simulink model "withshapingprgmdistsim"  (Simulink 6.3)
settings: Solver=ode45  StartTime=0.0  StopTime=60  RelTol=1e-3
values from neighbouring files (symbols this model uses):
  A = [  -0.1778         0         0         0         0   -9.7807   -9.7807 ... (first row only)    [shapingprgmdist.m]    (also in shapingprgmdist_withsigma.m)
  Aw = [-1/tauc 0; 0 -1/tauc]    [shapingprgmdist.m]    (also in shapingprgmdist_withsigma.m)
  B = [B1(:,1) B1(:,2) B1(:,4)]    [shapingprgmdist.m]    (also in shapingprgmdist_withsigma.m)
  Bw = .5*eye(2)    [shapingprgmdist.m]    (also in shapingprgmdist_withsigma.m)
  C = zeros(5,11)    [shapingprgmdist.m]    (also in shapingprgmdist_withsigma.m)
  D = [(W1G.a(:,1)) (W1G.a(:,2))]    [shapingprgmdist.m]    (also in shapingprgmdist_withsigma.m)
  den11 = [1 5 0]    [shapingprgmdist.m]    (also in shapingprgmdist_withsigma.m)
  den22 = den11    [shapingprgmdist.m]    (also in shapingprgmdist_withsigma.m)
  den33 = den11    [shapingprgmdist.m]    (also in shapingprgmdist_withsigma.m)
  K = inv(R)*(B'*P)*C'*inv(C*C')    [Hinfopfb.m]    (also in shapingprgmdist.m = Hinfopfb(W1G.a,W1G.b,W1G.c,D,gamma,Q,R); shapingprgmdist_withsigma.m = Hinfopfb(W1G.a,W1G.b,W1G.c,D,gamma,Q,R))
  num11 = 3*[1 0.5]    [shapingprgmdist.m]    (also in shapingprgmdist_withsigma.m)
  num22 = num11    [shapingprgmdist.m]    (also in shapingprgmdist_withsigma.m)
  num33 = num11    [shapingprgmdist.m]    (also in shapingprgmdist_withsigma.m)
  Phicorr = 1    [shapingprgmdist.m]    (also in shapingprgmdist_withsigma.m)
  qu = -20*0.3048    (= -6.096)    [shapingprgmdist.m]    (also in shapingprgmdist_withsigma.m)
  qv = -20*0.3048    (= -6.096)    [shapingprgmdist.m]    (also in shapingprgmdist_withsigma.m)
  Thetacorr = 1    [shapingprgmdist.m]    (also in shapingprgmdist_withsigma.m)
  W2 = diag([1 1 1 1 1])    [shapingprgmdist.m]    (also in shapingprgmdist_withsigma.m)
libraries: simulink x1
settings Model: LastModifiedBy=JG

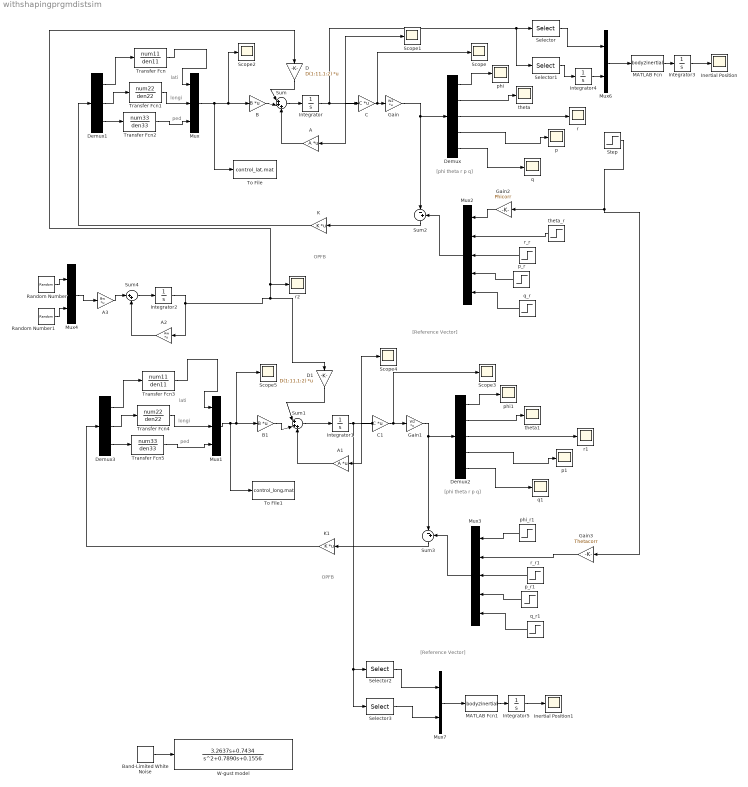
== system withshapingprgmdistsim ==
  note: OPFB
  note: [phi theta r p q]
  note: lati
  note: longi
  note: ped
  note: [Reference Vector]
  note: OPFB
  note: [phi theta r p q]
  note: [Reference Vector]
  note: lati
  note: longi
  note: ped
  A : Gain  Orientation=left  Gain=A  Multiplication=Matrix(K*u)
  A1 : Gain  Orientation=left  Gain=A  Multiplication=Matrix(K*u)
  A2 : Gain  Orientation=left  Gain=Aw  Multiplication=Matrix(K*u)
  A3 : Gain  Gain=Bw  Multiplication=Matrix(K*u)
  B : Gain  Gain=B  Multiplication=Matrix(K*u)
  B1 : Gain  Gain=B  Multiplication=Matrix(K*u)
  Band-Limited White Noise : simulink/Sources/Band-Limited White Noise  Cov=.1  Ts=0.1  seed=[23341]
  C : Gain  Gain=C  Multiplication=Matrix(K*u)
  C1 : Gain  Gain=C  Multiplication=Matrix(K*u)
  D : Gain  Orientation=down  Gain=D(1:11,1:2)  Multiplication=Matrix(K*u)
  D1 : Gain  Orientation=down  Gain=D(1:11,1:2)  Multiplication=Matrix(K*u)
  Demux : Demux  Outputs=5
  Demux1 : Demux  Outputs=3
  Demux2 : Demux  Outputs=5
  Demux3 : Demux  Outputs=3
  Gain : Gain  Gain=W2  Multiplication=Matrix(K*u)
  Gain1 : Gain  Gain=W2  Multiplication=Matrix(K*u)
  Gain2 : Gain  Orientation=left  Gain=Phicorr
  Gain3 : Gain  Orientation=left  Gain=Thetacorr
  Inertial Position : Scope
      settings: SaveName=InertialPos  DataFormat=Array
  Inertial Position1 : Scope
      settings: SaveName=InertialPos1  DataFormat=Array
  Integrator : Integrator  InitialCondition=rand((size(A,1)),1)*0.01
  Integrator1 : Integrator  InitialCondition=rand((size(A,1)),1)*0.01
  Integrator2 : Integrator
  Integrator3 : Integrator  InitialCondition=[0;0;-50]
  Integrator4 : Integrator
  Integrator5 : Integrator  InitialCondition=[0;0;-50]
  K : Gain  Orientation=left  Gain=K  Multiplication=Matrix(K*u)
  K1 : Gain  Orientation=left  Gain=K  Multiplication=Matrix(K*u)
  MATLAB Fcn : MATLABFcn  MATLABFcn=body2inertial
  MATLAB Fcn1 : MATLABFcn  MATLABFcn=body2inertial
  Mux : Mux  Inputs=3
  Mux1 : Mux  Inputs=3
  Mux2 : Mux  Orientation=left  Inputs=5
  Mux3 : Mux  Orientation=left  Inputs=5
  Mux4 : Mux  Inputs=2
  Mux6 : Mux  Inputs=2
  Mux7 : Mux  Inputs=2
  Random Number : RandomNumber  Variance=qu^2  SampleTime=0
  Random Number1 : RandomNumber  Variance=qv^2  Seed=5000  SampleTime=0
  Scope{,1..5} (6 alike) : Scope
      Scope settings: SaveName=y  DataFormat=Array
      Scope1 settings: SaveName=x1  DataFormat=Array
      Scope2 settings: SaveName=ScopeData8
      Scope3 settings: SaveName=y2  DataFormat=Array
      Scope4 settings: SaveName=x2  DataFormat=Array
  Selector : Selector  Elements=[1 2 9 5 6]  InputPortWidth=11
  Selector1 : Selector  Elements=[10]  InputPortWidth=11
  Selector2 : Selector  Elements=[1 2 9 5 6]  InputPortWidth=11
  Selector3 : Selector  Elements=10  InputPortWidth=11
  Step : Step  Time=0  SampleTime=0
  Sum : Sum  Inputs=|+++
  Sum1 : Sum  Inputs=|+++
  Sum2 : Sum  Orientation=down  Inputs=|-+
  Sum3 : Sum  Orientation=down  Inputs=|-+
  Sum4 : Sum  Inputs=|++
  To File : ToFile  Filename=control_lat.mat  MatrixName=ulat
  To File1 : ToFile  Filename=control_long.mat  MatrixName=ulong
  Transfer Fcn : TransferFcn  Numerator=num11  Denominator=den11
  Transfer Fcn1 : TransferFcn  Numerator=num22  Denominator=den22
  Transfer Fcn2 : TransferFcn  Numerator=num33  Denominator=den33
  Transfer Fcn3 : TransferFcn  Numerator=num11  Denominator=den11
  Transfer Fcn4 : TransferFcn  Numerator=num22  Denominator=den22
  Transfer Fcn5 : TransferFcn  Numerator=num33  Denominator=den33
  W-gust model : TransferFcn  Numerator="[3.2637    0.7434]"  Denominator="[1.0000    0.7890    0.1556]"
  p : Scope
      settings: SaveName=ScopeData4
  p1 : Scope
      settings: SaveName=ScopeData6
  p_r : Step  Orientation=left  Time=0  After=0  SampleTime=0
  p_r1 : Step  Orientation=left  Time=0  After=0  SampleTime=0
  phi : Scope
  phi1 : Scope
      settings: SaveName=ScopeData7
  phi_r1 : Step  Orientation=left  Time=0  After=0  SampleTime=0
  q : Scope
      settings: SaveName=ScopeData5
  q1 : Scope
      settings: SaveName=ScopeData9
  q_r : Step  Orientation=left  Time=0  After=0  SampleTime=0
  q_r1 : Step  Orientation=left  Time=0  After=0  SampleTime=0
  r : Scope
      settings: SaveName=ScopeData3
  r1 : Scope
      settings: SaveName=ScopeData10
  r2 : Scope
      settings: SaveName=d  DataFormat=Array
  r_r : Step  Orientation=left  Time=0  After=0  SampleTime=0
  r_r1 : Step  Orientation=left  Time=0  After=0  SampleTime=0
  theta : Scope
      settings: SaveName=ScopeData2
  theta1 : Scope
      settings: SaveName=ScopeData11
  theta_r : Step  Orientation=left  Time=0  After=0  SampleTime=0
  wires:
  Integrator/1 -> A/1, C/1, Scope1/1, Selector/1, Selector1/1
  Sum/1 -> Integrator/1
  C/1 -> Gain/1, Scope/1
  Mux/1 -> B/1, Scope2/1, To File/1
  Mux2/1 -> Sum2/2
  r_r/1 -> Mux2/3
  Sum2/1 -> K/1
  K/1 -> Demux1/1
  Demux/1 -> phi/1
  Demux/2 -> theta/1
  Demux/3 -> r/1
  Step/1 -> Gain2/1, Gain3/1
  theta_r/1 -> Mux2/2
  p_r/1 -> Mux2/4
  q_r/1 -> Mux2/5
  Demux/4 -> p/1
  Demux/5 -> q/1
  Integrator1/1 -> A1/1, C1/1, Scope4/1, Selector3/1, Selector2/1
  Sum1/1 -> Integrator1/1
  C1/1 -> Gain1/1, Scope3/1
  Mux1/1 -> B1/1, Scope5/1, To File1/1
  Mux3/1 -> Sum3/2
  r_r1/1 -> Mux3/3
  Sum3/1 -> K1/1
  K1/1 -> Demux3/1
  Demux2/1 -> phi1/1
  Demux2/2 -> theta1/1
  Demux2/3 -> r1/1
  phi_r1/1 -> Mux3/1
  p_r1/1 -> Mux3/4
  q_r1/1 -> Mux3/5
  Demux2/4 -> p1/1
  Demux2/5 -> q1/1
  Demux1/1 -> Transfer Fcn/1
  Demux1/3 -> Transfer Fcn2/1
  Demux1/2 -> Transfer Fcn1/1
  Transfer Fcn1/1 -> Mux/2
  Demux3/1 -> Transfer Fcn3/1
  Demux3/3 -> Transfer Fcn5/1
  Transfer Fcn5/1 -> Mux1/3
  Demux3/2 -> Transfer Fcn4/1
  Transfer Fcn4/1 -> Mux1/2
  Gain/1 -> Demux/1, Sum2/1
  Gain1/1 -> Demux2/1, Sum3/1
  Transfer Fcn2/1 -> Mux/3
  Gain2/1 -> Mux2/1
  Gain3/1 -> Mux3/2
  A/1 -> Sum/3
  B/1 -> Sum/2
  A1/1 -> Sum1/3
  B1/1 -> Sum1/2
  Transfer Fcn3/1 -> Mux1/1
  Transfer Fcn/1 -> Mux/1
  D/1 -> Sum/1
  D1/1 -> Sum1/1
  Band-Limited White Noise/1 -> W-gust model/1
  Integrator2/1 -> A2/1, D1/1, D/1, r2/1
  Random Number/1 -> Mux4/1
  Random Number1/1 -> Mux4/2
  A2/1 -> Sum4/2
  Sum4/1 -> Integrator2/1
  Mux4/1 -> A3/1
  A3/1 -> Sum4/1
  Mux6/1 -> MATLAB Fcn/1
  MATLAB Fcn/1 -> Integrator3/1
  Selector/1 -> Mux6/1
  Integrator4/1 -> Mux6/2
  Selector1/1 -> Integrator4/1
  Integrator3/1 -> Inertial Position/1
  Mux7/1 -> MATLAB Fcn1/1
  MATLAB Fcn1/1 -> Integrator5/1
  Selector2/1 -> Mux7/1
  Integrator5/1 -> Inertial Position1/1
  Selector3/1 -> Mux7/2
